simulink model "model_7"  (R2020a)
settings: Solver=VariableStepAuto  StartTime=0.0  StopTime=10.0  RelTol=1e-3
settings Model: Creator=Notnik_kg  LastModifiedBy=Notnik_kg

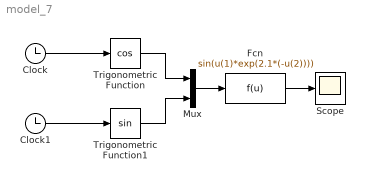
== system model_7 ==
  Clock : Clock
  Clock1 : Clock
  Fcn : Fcn  Expr=sin(u(1)*exp(2.1*(-u(2))))
  Mux : Mux  Inputs=2
  Scope : Scope
  Trigonometric Function : Trigonometry  Operator=cos
  Trigonometric Function1 : Trigonometry
  wires:
  Clock1/1 -> Trigonometric Function1/1
  Clock/1 -> Trigonometric Function/1
  Mux/1 -> Fcn/1
  Fcn/1 -> Scope/1
  Trigonometric Function/1 -> Mux/1
  Trigonometric Function1/1 -> Mux/2
